simulink library "SignalOverride"  (R2022b)
settings: Solver=VariableStepAuto  StartTime=0.0  StopTime=10.0  RelTol=1e-3
libraries: FeaturePath x1, RTC x1
settings Model: Creator=kl13806  LastModifiedBy=kl13806
settings SolverCC: AlgebraicLoopSolver=TrustRegion
settings DebuggingCC: UnconnectedInputMsg=warning  UnconnectedOutputMsg=warning  UnconnectedLineMsg=warning  SFMachineParentedDataDiag=warning  ArithmeticOperatorsInVariantConditions=warning
settings ModelReferenceCC: EnableRefExpFcnMdlSchedulingChecks=on
settings SFSimCC: SimUseLocalCustomCode=off  CustomCodeUndefinedFunction=UseInterfaceOnly
settings RTWCC: RTWUseLocalCustomCode=off  DLArmComputeVersion=19.05
settings CodeAppCC: StateflowObjectComments=on

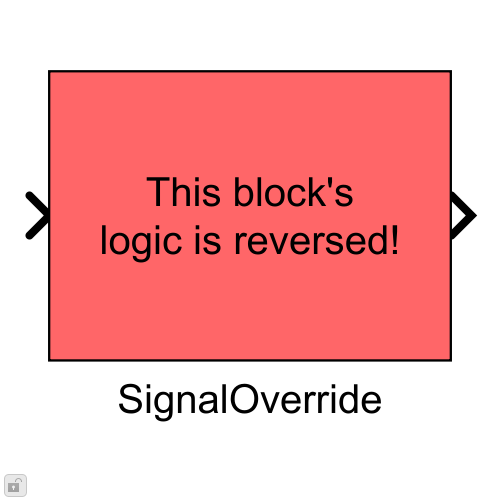
[thumbnail: Simulink's stored preview of the top-level diagram]
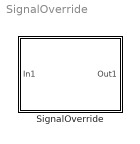
== system SignalOverride ==
  SignalOverride : Subsystem  mask(Bose Signal Override){MaskSignalName=, MaskDataTypeStr=single, MaskSignalWidth=1, LastName=, TriggerInit=[35 19 135 91]}
      mask prompts: MaskSignalName "Signal Name"; MaskDataTypeStr "Signal Type"; MaskSignalWidth "Signal Width"; LastName "non-visible helper to detect name change"; TriggerInit "Hidden: MoveFcn redraw"
      mask help: This creates the ability to override a signal at runtime. Only scalar and vector signals are currently supported (too lazy to put a reshaper block in there).
      mask init:
      | theSID = Simulink.ID.getSID(gcbh);
      | [ok] = SignalOverrideMask.Init(gcbh);
      | 
      | % This block has reversed logic in terms of when the override is applied...
      | % and yet it's been lingering around for years without correction. Possibly
      | % some projects are using it anyway and just flipping the logic someplace
      | % else so it "works". As automatically correcting this defect seems
      | % dangerous, instead a new corrected block is added and the below warning
      | % may enable people to click a link to replace the original bad block with
      | % the new good one... and of course make sure to undo whatever reversals
      | % they already have in place for that project.
      | goodBlock = 'OverrideSignal/OverrideSignal';
      | if (false == strcmp(theSID,'SignalOverride:1'))
      |     warning(['The SignalOverride block has reversed logic! ' ...
      |         'If you are using this block, perhaps the logic is switched ' ...
      |         'elsewhere to correct it?! A recipe for disaster. Please replace ', ...
      |         'with the corrected "OverrideSignal" block and correct the integration ' ...
      |         'logic to no longer be reversed. This link will replace the block ' ...
      |         'but emit a few errors about LastName and TriggerInit: ' ...
      |         '<a href="matlab:set_param(''%s'',''ReferenceBlock'',''%s'')">FIX IT</a>'], ...
      |     theSID,goodBlock);
      | end
      settings: MoveFcn=SignalOverrideMask.CB_TriggerInit(gcbh);
      mask TypeOptions MaskSignalName: FeaturePath/FeatureName
      mask TypeOptions MaskDataTypeStr: RTC Override/REQElemType2
      mask TypeOptions MaskSignalWidth: RTC Override/REQElemWidth2
      mask Callback TriggerInit: SignalOverrideMask.CB_TriggerInit(gcbh);
      mask DialogControl ErrorContainer Prompt: Error Messages
      mask Display: disp("This block's\nlogic is reversed!")

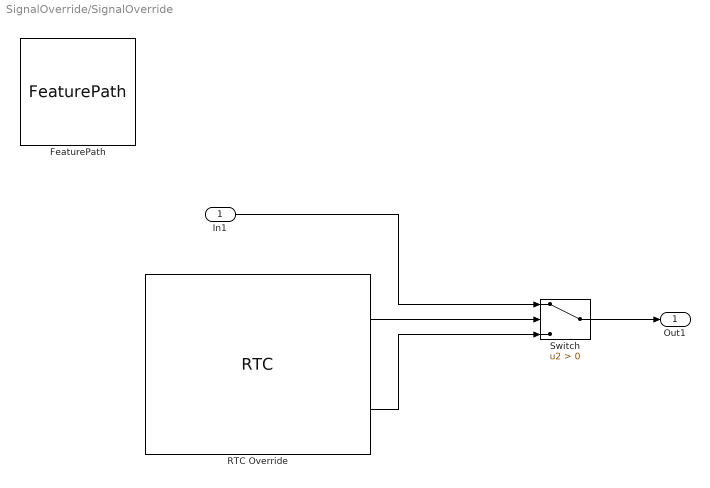
== system SignalOverride/SignalOverride ==
  In1 : Inport
  FeaturePath : FeaturePath/FeaturePath  IsGroup=off  GroupNumber=-1  IsModule=off  TriggerInit=[265 104 380 211]
  RTC Override : RTC/RTC  Description=Enables a signal to be overridden by a runtime request (RTC).  REQ_Priority=RTC_Mask.NormalPriority  RequestAtInit=off  EnableRequest=off  REQElemName1=enable_override  REQElemType1=uint32  REQElemWidth1=1  REQElemInitial1=[]  REQElemName2=override_value  REQElemType2=single  REQElemWidth2=MaskSignalWidth  REQElemInitial2=[]  REQElemType3=uint32  REQElemWidth3=1  REQElemInitial3=[]  REQElemType4=uint32  REQElemWidth4=1  REQElemInitial4=[]  REQElemType5=uint32  REQElemWidth5=1  REQElemInitial5=[]  REQElemType6=uint32  REQElemWidth6=1  REQElemInitial6=[]  REQElemType7=uint32  REQElemWidth7=1  REQElemInitial7=[]  REQElemType8=uint32  REQElemWidth8=1  REQElemInitial8=[]  REQElemType9=uint32  REQElemWidth9=1  REQElemInitial9=[]  REQElemType10=uint32  REQElemWidth10=1  REQElemInitial10=[]  EnableResponse=off  EnableRSP_StatusIn=off  RSPElemType1=uint32  RSPElemWidth1=1  RSPElemType2=uint32  RSPElemWidth2=1  RSPElemType3=uint32  RSPElemWidth3=1  RSPElemType4=uint32  RSPElemWidth4=1  RSPElemType5=uint32  RSPElemWidth5=1  RSPElemType6=uint32  RSPElemWidth6=1  RSPElemType7=uint32  RSPElemWidth7=1  RSPElemType8=uint32  RSPElemWidth8=1  RSPElemType9=uint32  RSPElemWidth9=1  RSPElemType10=uint32  RSPElemWidth10=1  EnableNotification=off  EnableNTF_PrepTrig=off  NTFElemType1=uint32  NTFElemWidth1=1  NTFElemType2=uint32  NTFElemWidth2=1  NTFElemType3=uint32  NTFElemWidth3=1  NTFElemType4=uint32  NTFElemWidth4=1  NTFElemType5=uint32  NTFElemWidth5=1  NTFElemType6=uint32  NTFElemWidth6=1  NTFElemType7=uint32  NTFElemWidth7=1  NTFElemType8=uint32  NTFElemWidth8=1  NTFElemType9=uint32  NTFElemWidth9=1  NTFElemType10=uint32  NTFElemWidth10=1  MaskMessageName=Override
  Switch : Switch  Criteria=u2 > Threshold  SaturateOnIntegerOverflow=off  InputSameDT=off
  Out1 : Outport  VectorParamsAs1DForOutWhenUnconnected=off
  wires:
  In1/1 -> Switch/1
  Switch/1 -> Out1/1
  RTC Override/2 -> Switch/3
  RTC Override/1 -> Switch/2
